simulink model "switch_bus_test"  (Simulink 8.4)
settings: Solver=FixedStepDiscrete  StartTime=0.0  StopTime=10.0  FixedStep=1.0  RelTol=1e-3
settings Model: Creator=arnaud  LastModifiedBy=arnaud
settings DataIOCC: SaveFormat=Structure
settings DebuggingCC: FcnCallInpInsideContextMsg=EnableAllAsError

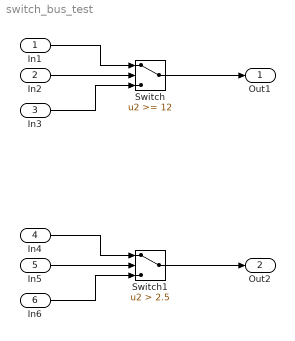
== system switch_bus_test ==
  In1 : Inport  OutDataTypeStr=Bus: BusA  BusOutputAsStruct=on
  In2 : Inport  Port=2  OutDataTypeStr=int8
  In3 : Inport  Port=3  OutDataTypeStr=Bus: BusA  BusOutputAsStruct=on
  In4 : Inport  Port=4  OutDataTypeStr=Bus: BusB  PortDimensions=1  BusOutputAsStruct=on
  In5 : Inport  Port=5  OutDataTypeStr=boolean  PortDimensions=1
  In6 : Inport  Port=6  OutDataTypeStr=Bus: BusB  PortDimensions=1  BusOutputAsStruct=on
  Switch : Switch  Threshold=12
  Switch1 : Switch  Criteria=u2 > Threshold  Threshold=2.5
  Out1 : Outport
  Out2 : Outport  Port=2
  wires:
  In1/1 -> Switch/1
  In2/1 -> Switch/2
  In3/1 -> Switch/3
  Switch/1 -> Out1/1
  In4/1 -> Switch1/1
  In5/1 -> Switch1/2
  In6/1 -> Switch1/3
  Switch1/1 -> Out2/1
